simulink model "stackedRotor_dualEMRAX_dynInflow"  (R2022b)
settings: Solver=ode45  StartTime=0.0  StopTime=60  RelTol=1e-4  EnableMultiTasking=on
InitFcn:
  | %Hide scope plots
  | HidHandles = get(0,'ShowHiddenHandles');
  | set(0,'ShowHiddenHandles','On');
  | AllScopeHandles = findobj(0,'Type','Figure','Tag','SIMULINK_SIMSCOPE_FIGURE');
  | close(AllScopeHandles);
  | set(0,'ShowHiddenHandles',HidHandles);
  | 
  | %Load Cl and Cd from potential flow
  | load('C:\Users\msa2925\Box\Matt Lab Stuff\5th Year\Modeling\Look Up Tables\ClCd-1.mat');
  | 
  | %Load dynamic inflow properties (model and rotor_params)
  | load('C:\Users\msa2925\Box\Matt Lab Stuff\5th Year\Modeling\Look Up Tables\DynInflow-1.mat');
  | 
  | 
  | %Atmospheric Properties
  | rho_air    = 1.225;  % air density in kg/m^3
  | mu         = 1.803e-5; % dynamic viscosity [N-s/m^2]
  | 
  | %Emrax 208 Electrical Properties
  | R          = .0122;  %  resistance, ohms, line-line at room temp
  | L          = 125*10^-6;  %  inductance line-line at commutation frequency, henries
  | t_elec     = L/R;
  | Imotor     = 256/100^2;  %  kg*m^2 -- From Emrax data sheet
  | Kt_motor   = .80;  %  N*m/Arms
  | Ke_motor   = .0487*sqrt(2)*60/(2*pi);  %  Vpk/rad/sec
  | Ke         = .0487*sqrt(2)*60/(2*pi);   %radians/sec
  | POLES      = 20;
  | 
  | % no-load current fit (i0 = a1*omega^2 + a2) [Apk]
  | i_a1 = 8.98e-5;
  | i_a2 = 2.51;
  | 
  | %-----------Controller Properties------------------%
  | Vbus                 = 175;  % Actual bus voltage (volts) that will be applied
  | CurrentSenseMax      = 250;  %  Max current sense from controller code
  | BASE_CURRENT         = 125;   %  Max current in amps corresponding to normalized control loop current = 1
  | LOOP_FREQUENCY       = 35;     % orig: 35 in kHz
  | T_LOOP               = .001/LOOP_FREQUENCY;
  | pwm_loop_prescalar   = 1;  %Presacalar how many PWM cycles for one current loop execution
  | T_PWM                = T_LOOP/pwm_loop_prescalar;  %  Current loop prescaler on PWM is 1 for Uber
  | BASE_FREQ            = 1200; %POLES/2*1300/60;  %  1300 rpm
  | BaseSpeed            = BASE_FREQ*(60.0/(POLES/2.0));
  | omega                = 0;               % omega for de-coupling integrator
  | MsgFreq              = 1000; %Hz
  | 
  | %Current loop
  | alpha    = 250*2*pi;         % current loop bandwidth
  | I_Kp     = alpha*L*1;
  | I_Ki     = alpha*R/I_Kp*T_LOOP;
  | 
  | %Speed loop
  | SpeedLoopPrescale  = 5;
  | Tspeedloop         = T_LOOP*SpeedLoopPrescale;
  | PID_spd_Kp         = 4.75;   % From Uber code (ORIGINIAL: 3)
  | % PID_spd_Ki         = 2.1*Tspeedloop*1.5;   % From Uber code (ORIGINAL: 0.15*Tspeedloop*2)
  | PID_spd_Ki         = 1.75*Tspeedloop;
  | 
  | %Position loop
  | speedErrorPEngage    = .003; % Speed error max for position loop to enable
  | % Code has .001 for PEngage, trying something diff here
  | ... (+44 lines)
values from neighbouring files (symbols this model uses):
  AoA_sweep = [-2 -1 0 1 2 3 4 5 6 7 8 9 ... (13 elements, 1x13)]    [ClCd-1.mat]
  Cdl = [0.0123 0.0123 0.0123 0.0123 0.0123 0.0123 0.0123 0.0123 0.0123 0.0123 0.0123 0.0123 ... (6500 elements, 13x500)]    [ClCd-1.mat]
  Cdu = [0.0123 0.0123 0.0123 0.0123 0.0123 0.0123 0.0123 0.0123 0.0123 0.0123 0.0123 0.0123 ... (6500 elements, 13x500)]    [ClCd-1.mat]
  Cll = [-0.111113403346 0.00796289645531 0.127036770682 0.246071948277 0.365032169973 0.483881199334 0.602582833794 0.721100915686 0.839399343253 0.957442081649 1.07519317391 1.19261675192 ... (6500 elements, 13x500)]    [ClCd-1.mat]
  Clu = [-0.11705321178 0.00839337636768 0.133837407812 0.259240671085 0.384564967138 0.509772120977 0.634823993289 0.759682492064 0.884309584192 1.00866730705 1.13271778008 1.2564232163 ... (6500 elements, 13x500)]    [ClCd-1.mat]
  Cp = [0.000195201118563 0.000195344815163 0.000195970524669 0.000196911243155 0.000198292722473 0.000199793715635 0.000201836164013 0.000204359459521 0.00020706119236 0.00020992934584 0.000212955219574 0.000216131124695 ... (150 elements, 1x150)]    [BEMT-1.mat]    (also in BEMT-2.mat = [5.908e-05 5.908e-05 5.908e-05 5.908e-05 5.908e-05 5.908e-05; BEMT-3.mat = [6.167e-05 6.167e-05 6.167e-05 6.167e-05 6.167e-05 6.1671725; BEMT-PF-Isolated-1.mat = [6.88284627296e-05 6.76929537705e-05 6.92283244838e-05 7.518; BEMT-PF-Isolated-2.mat = [6.88286203447e-05 6.76929720507e-05 6.92293837373e-05 7.518)
  Cpl = [0.000333700998998 0.000390181039031 0.000394788670278 0.000400729506228 0.000408611755119 0.000419410254194 0.000434611180529 0.000454621522012 0.000471293145772 0.000468819202162 0.000461044856051 0.0004465872684 ... (37 elements, 1x37)]    [BEMT-PF-Stacked-1.mat]    (also in BEMT-PF-Stacked-3.mat = [0.00012095698162 0.000162284223538 0.000164817714818 0.0001; BEMT-PF-Stacked-4.mat = [0.000215313097577 0.00022323140747 0.000225181363314 0.0002; BEMT-PF-Stacked-5.mat = [0.000201399004141 0.000209364989981 0.000211223578331 0.000; CpData-Stacked-1.mat = [0.0004204989393 0.000429722690454 0.000432518606247 0.00043)
  Cpu = [0.000372640330495 0.000318761476241 0.00031503993434 0.000310316169544 0.000304143730405 0.000295773643033 0.00028387117424 0.000265492168428 0.000237641915024 0.000230728320611 0.000223594040333 0.000216887343718 ... (37 elements, 1x37)]    [BEMT-PF-Stacked-1.mat]    (also in BEMT-PF-Stacked-3.mat = [0.00014995136179 0.000108984048023 0.00010569458686 0.00010; BEMT-PF-Stacked-4.mat = [0.000200079302516 0.0001931098957 0.000191441123461 0.00018; BEMT-PF-Stacked-5.mat = [0.000223261524278 0.000214635121691 0.000212581398187 0.000; CpData-Stacked-1.mat = [0.000470292570894 0.000463315827435 0.000462372188797 0.000)
  Ct = [0 8.42066058624e-05 0.000168413211725 0.000252619817587 0.000348569118235 0.000435711397794 0.000522853677352 0.000609995956911 0.00069713823647 0.000784280516029 0.000871422795587 0.000958565075146 ... (150 elements, 1x150)]    [BEMT-1.mat]    (also in BEMT-2.mat = [-0.000241284312952 -0.00019885713846 -0.000156429963968 -0.; BEMT-3.mat = [-0.000252881464423 -0.00020500571035 -0.00015767832519 -0.0; BEMT-PF-Isolated-1.mat = [-0.000124730397385 6.78902114512e-07 0.000152796242494 0.00; BEMT-PF-Isolated-2.mat = [-0.000124743531158 6.68801957239e-07 0.000152879013625 0.00)
  Ctl = [0.00438668608339 0.0050628698524 0.00511522584539 0.00518172746808 0.00526807639226 0.00538256546486 0.00553531477508 0.00571551109899 0.00580582681419 0.00575766596858 0.00565748394784 0.00549586936617 ... (37 elements, 1x37)]    [BEMT-PF-Stacked-1.mat]    (also in BEMT-PF-Stacked-2.mat = [0.00446656952376 0.00504151525843 0.00508284852112 0.005134; BEMT-PF-Stacked-3.mat = [0.00184996435909 0.00209589101081 0.00210506301257 0.002127; BEMT-PF-Stacked-4.mat = [0.00305779502317 0.00317485141984 0.00320289061972 0.003237; BEMT-PF-Stacked-5.mat = [0.00284078729023 0.00295761000687 0.00298453442892 0.003017)
  Ctu = [0.00485875244254 0.00420098979139 0.00415434112966 0.00409491081367 0.00401692201007 0.00391066006909 0.00375881977479 0.00352379292731 0.0031675839941 0.00307949239151 0.00298865074931 0.00290335167779 ... (37 elements, 1x37)]    [BEMT-PF-Stacked-1.mat]    (also in BEMT-PF-Stacked-2.mat = [0.00487929290239 0.00430977798758 0.00426987840094 0.004219; BEMT-PF-Stacked-3.mat = [0.00202552929257 0.00178155832272 0.00175724958711 0.001735; BEMT-PF-Stacked-4.mat = [0.00282403441036 0.00271496837402 0.00268870985611 0.002655; BEMT-PF-Stacked-5.mat = [0.00315608603824 0.00303364263049 0.00300412792098 0.002966)
  index_sweep = [-90 -45 -40 -35 -30 -25 -20 -15 -10 -9 -8 -7 ... (37 elements, 1x37)]    [BEMT-PF-Stacked-1.mat]    (also in BEMT-PF-Stacked-2.mat; BEMT-PF-Stacked-3.mat = [-90 -45 -40 -35 -30 -25 -20 -15 -14 -13 -12 -11 ... (45 ele; BEMT-PF-Stacked-4.mat; BEMT-PF-Stacked-5.mat)
  index_sweep_Cp_table = [-90 -45.2679945682 -41.0748847617 -35.9788199136 -30.8261561384 -25.6873115637 -20.5477936424 -15.3629851439 -10.3005197032 -7.23856497031 -5.29357093665 -4.47027434572 ... (27 elements, 1x27)]    [CpData-Stacked-1.mat]
  model =     [DynInflow-1.mat]    (also in PP-1.mat; PP-2.mat; PP-3.mat)
  rotor_params =     [DynInflow-1.mat]    (also in PP-1.mat; PP-2.mat; PP-3.mat)
  theta = [-1.24244156171 -0.730247869575 -0.489791195362 -0.291308360013 -0.0904887039498 0.0775201787218 0.236938510902 0.389966557012 0.537998944025 0.680941129328 0.820002111662 0.955737387113 ... (150 elements, 1x150)]    [BEMT-1.mat]    (also in BEMT-2.mat = [-2.67472972391 -2.52181622329 -2.35655527709 -2.17339529035; BEMT-3.mat = [-2.61565298703 -2.45920727031 -2.29202818901 -2.11251263407; BEMT-PF-Isolated-1.mat = [-2 -1 0 1 2 3 4 5 6 7 8 9 ... (16 elements, 1x16)]; BEMT-PF-Isolated-2.mat = [-2 -1 0 1 2 3 4 5 6 7 8 9 ... (16 elements, 1x16)])
  x_sweep = [-1.74044233009 -1.73346660933 -1.72649088856 -1.7195151678 -1.71253944704 -1.70556372628 -1.69858800552 -1.69161228476 -1.68463656399 -1.67766084323 -1.67068512247 -1.66370940171 ... (500 elements, 1x500)]    [ClCd-1.mat]
undefined symbols (not defined in the file or in its folder): DiscIntNeverNeededParam
libraries: dspsrcs4 x2
(part 2 of 2)

== system stackedRotor_dualEMRAX_dynInflow/Follower/SVGEN-PWM ==
  note: Saturate to complex magnitude 1
  note: Output to PWM
      | after 11 us compute time
      | and wait for new PWM start
  note: Average V
      | across winding
      | takes 1 PWM
      | cycle to happen
  note: Compute
      | me
  DQ V : Inport
  Bus Voltage : Inport  Port=2
  Avg PWM voltage in DQ space : Product  RndMeth=Zero
  Complex to Magnitude-Angle : ComplexToMagnitudeAngle
  Complex to Real-Imag : ComplexToRealImag
  Conv to Cont time for Electical stuff : RateTransition
  Demux : Demux  Outputs=2
  Divide : Product  Inputs=/*
  Gain1 : Gain  Gain=1/sqrt(3)
  Into SVGEN : UnitDelay  InitialCondition=[ 0 ; omegamech*Ke/Vbus]  SampleTime=-1
  Magnitude-Angle to Complex : MagnitudeAngleToComplex
  Measure Bus V ADC : RateTransition  OutPortSampleTime=T_LOOP
  Mux : Mux  Inputs=2
  PWM emulation : RateTransition  OutPortSampleTime=T_PWM
  Real-Imag to Complex : RealImagToComplex
  Saturation : Saturate  UpperLimit=1  LowerLimit=-1
  Unit Delay : UnitDelay  InitialCondition=[ 0 ; omegamech*Ke/Vbus]  SampleTime=-1
  Unit Delay2 : UnitDelay  InitialCondition=[ 0 ; omegamech*Ke/Vbus]  SampleTime=-1
  DQ Volts : Outport
  wires:
  Into SVGEN/1 -> PWM emulation/1
  Unit Delay/1 -> Unit Delay2/1
  PWM emulation/1 -> Unit Delay/1
  Unit Delay2/1 -> Conv to Cont time for Electical stuff/1
  Bus Voltage/1 -> Gain1/1
  Measure Bus V ADC/1 -> Divide/1
  DQ V/1 -> Divide/2
  Conv to Cont time for Electical stuff/1 -> Avg PWM voltage in DQ space/2
  Avg PWM voltage in DQ space/1 -> DQ Volts/1
  Mux/1 -> Into SVGEN/1
  Divide/1 -> Demux/1
  Demux/1 -> Real-Imag to Complex/1
  Demux/2 -> Real-Imag to Complex/2
  Real-Imag to Complex/1 -> Complex to Magnitude-Angle/1
  Complex to Magnitude-Angle/1 -> Saturation/1
  Saturation/1 -> Magnitude-Angle to Complex/1
  Complex to Magnitude-Angle/2 -> Magnitude-Angle to Complex/2
  Magnitude-Angle to Complex/1 -> Complex to Real-Imag/1
  Complex to Real-Imag/1 -> Mux/1
  Complex to Real-Imag/2 -> Mux/2
  Gain1/1 -> Measure Bus V ADC/1, Avg PWM voltage in DQ space/1

== system stackedRotor_dualEMRAX_dynInflow/Follower/Speed Control? ==
  In1 : Inport
  Abs : Abs  SaturateOnIntegerOverflow=off
  Relay : Relay  OnSwitchValue=2*speedErrorPEngage  OffSwitchValue=speedErrorPEngage  OnOutputValue=0  OffOutputValue=1
  Out1 : Outport
  wires:
  Abs/1 -> Relay/1
  In1/1 -> Abs/1
  Relay/1 -> Out1/1

== system stackedRotor_dualEMRAX_dynInflow/Follower/Speed Controller ==
  In1 : Inport
  Initial Cond : Inport  Port=2
  Enable : EnablePort  ShowOutputPort=on
  1/integraltime to match code since Simulink integrator has Ts term : Gain  Gain=1/(T_LOOP*SpeedLoopPrescale)
  Add1 : Sum
  ControllerIN : Scope
  Discrete-Time Integrator : DiscreteIntegrator  InitialCondition=.03  SampleTime=-1  ICPrevOutput=DiscIntNeverNeededParam  ICPrevScaledInput=DiscIntNeverNeededParam
  Integrator term at the output : Gain  Gain=PID_spd_Kp
  Product : Product  RndMeth=Zero
  Product1 : Product  RndMeth=Zero
  Speed I gain : Constant  Value=PID_spd_Ki
  Speed P gain : Constant  Value=PID_spd_Kp
  Out1 : Outport
  State : Outport  Port=2
  wires:
  Product/1 -> 1/integraltime to match code since Simulink integrator has Ts term/1
  In1/1 -> Product/1, Add1/1
  1/integraltime to match code since Simulink integrator has Ts term/1 -> Discrete-Time Integrator/1
  Speed I gain/1 -> Product/2
  Speed P gain/1 -> Product1/1
  Discrete-Time Integrator/1 -> Integrator term at the output/1, ControllerIN/1, Add1/2
  Add1/1 -> Product1/2
  Product1/1 -> Out1/1
  Integrator term at the output/1 -> State/1

== system stackedRotor_dualEMRAX_dynInflow/Follower/Speed Estimator ==
  In1 : Inport
  Add1 : Sum  Inputs=+-
  DeltaAngle : Scope
  Sampling : UnitDelay  SampleTime=-1
  Speed Estimator : Subsystem
  Unit Delay1 : UnitDelay  SampleTime=-1
  Out1 : Outport
  wires:
  Sampling/1 -> Add1/1, Unit Delay1/1
  Unit Delay1/1 -> Add1/2
  Add1/1 -> Speed Estimator/1(delta angle), DeltaAngle/1
  In1/1 -> Sampling/1
  Speed Estimator/1(Est Speed [0,1]) -> Out1/1

== system stackedRotor_dualEMRAX_dynInflow/Follower/Wrap error2 ==
  In1 : Inport
  Add 2pi : Subsystem  TreatAsAtomicUnit=on
  If Action Subsystem : Subsystem  TreatAsAtomicUnit=on
  If1 : If  IfExpression=u1 > .5  ElseIfExpressions=u1<-.5
  Merge : Merge  Inputs=3
  Subtract 2pi1 : Subsystem  TreatAsAtomicUnit=on
  Out1 : Outport
  wires:
  In1/1 -> Add 2pi/1(In1), If Action Subsystem/1(In1), Subtract 2pi1/1(In1), If1/1
  Subtract 2pi1/1(Out1) -> Merge/1
  Merge/1 -> Out1/1
  If1/1 -> Subtract 2pi1/Action
  If1/3 -> If Action Subsystem/Action
  Add 2pi/1(Out1) -> Merge/2
  If Action Subsystem/1(Out1) -> Merge/3
  If1/2 -> Add 2pi/Action

== system stackedRotor_dualEMRAX_dynInflow/Servo/Angle Controller ==
  In1 : Inport
  Initial Cond : Inport  Port=2
  Enable1 : Inport  Port=3
  Angle Controller DT_PID saturate P : Subsystem
  Max error : Saturate  UpperLimit=PID_pos_error_sat  LowerLimit=-PID_pos_error_sat
  Out1 : Outport  InitialOutput=[0]
  State : Outport  Port=2  InitialOutput=[0]
  wires:
  Initial Cond/1 -> Angle Controller DT_PID saturate P/2(Iniitial Cond)
  Enable1/1 -> Angle Controller DT_PID saturate P/Enable
  Angle Controller DT_PID saturate P/1(Out1) -> Out1/1
  Angle Controller DT_PID saturate P/2(Integrator) -> State/1
  In1/1 -> Max error/1
  Max error/1 -> Angle Controller DT_PID saturate P/1(In1)

== system stackedRotor_dualEMRAX_dynInflow/Servo/Angle Error ==
  Revolution : Inport
  Commanded Rev : Inport  Port=2
  Add4 : Sum  Inputs=-+
  Angle Error Calc Deg : Scope
  Gain2 : Gain  Gain=360
  To Workspace3 : ToWorkspace  VariableName=Angle_err_servo  SaveFormat=Timeseries  SampleTime=-1
  Wrap error : Subsystem
  Revolution Error (norm) : Outport
  tag scope: angle_err_servo=global
  wires:
  Revolution/1 -> Add4/1
  Wrap error/1(Out1) -> [angle_err_servo], Revolution Error (norm)/1, Gain2/1
  Gain2/1 -> To Workspace3/1, Angle Error Calc Deg/1
  Add4/1 -> Wrap error/1(In1)
  Commanded Rev/1 -> Add4/2

== system stackedRotor_dualEMRAX_dynInflow/Servo/Current Controller ==
  note: D Current Reference
  note: D Current Feedback
  note: D Current Reference
  note: Q Current Reference
  note: Discrete
      | time control
      | law
  QI cmd : Inport
  DQ I feedback : Inport  Port=2
  Constant : Constant  Value=0
  Constant1 : Constant  Value=0
  D current PI controller : Subsystem
  Decoupling gain : Gain  Gain=alpha*omega*L
  Decoupling gain1 : Gain  Gain=alpha*omega*L
  Demux : Demux  Outputs=2
  Discrete-Time Integrator : DiscreteIntegrator  SampleTime=T_LOOP  ICPrevOutput=DiscIntNeverNeededParam  ICPrevScaledInput=DiscIntNeverNeededParam
  Discrete-Time Integrator1 : DiscreteIntegrator  SampleTime=T_LOOP  ICPrevOutput=DiscIntNeverNeededParam  ICPrevScaledInput=DiscIntNeverNeededParam
  Manual Switch : ManualSwitch
  Manual Switch1 : ManualSwitch  CurrentSetting=0
  Mux1 : Mux  Inputs=2
  Q current PI controller : Subsystem
  Sum2 : Sum  Inputs=|+-
  Sum3 : Sum  Inputs=|+-
  Sum5 : Sum  Inputs=|+-
  Sum6 : Sum  Inputs=++|
  DQ V cmd : Outport
  wires:
  Mux1/1 -> DQ V cmd/1
  Sum2/1 -> D current PI controller/1(In1), Manual Switch1/1
  Sum3/1 -> Q current PI controller/1(In1), Manual Switch/2
  Constant/1 -> Sum2/1
  D current PI controller/1(Out1) -> Sum5/1
  Q current PI controller/1(Out1) -> Sum6/2
  Discrete-Time Integrator/1 -> Sum6/1
  Discrete-Time Integrator1/1 -> Sum5/2
  QI cmd/1 -> Sum3/1
  Decoupling gain1/1 -> Discrete-Time Integrator1/1
  Decoupling gain/1 -> Discrete-Time Integrator/1
  Manual Switch/1 -> Decoupling gain1/1
  Manual Switch1/1 -> Decoupling gain/1
  Constant1/1 -> Manual Switch1/2, Manual Switch/1
  Sum5/1 -> Mux1/1
  Sum6/1 -> Mux1/2
  DQ I feedback/1 -> Demux/1
  Demux/1 -> Sum2/2
  Demux/2 -> Sum3/2

== system stackedRotor_dualEMRAX_dynInflow/Servo/Generate Angle vs time ==
  Speed : Inport
  Phase (norm) : Inport  Port=2
  Add5 : Sum
  Constant1 : Constant
  Constant3 : Constant
  Discrete-Time Integrator : DiscreteIntegrator  SampleTime=-1  ICPrevOutput=DiscIntNeverNeededParam  ICPrevScaledInput=DiscIntNeverNeededParam
  Normalized Mech Angle : Gain  Gain=BASE_FREQ/(POLES/2)
  Wrap command : Math  Operator=mod  SignedPower=on
  Wrap command1 : Math  Operator=mod  SignedPower=on
  Cmd Angle (norm) : Outport
  Reference Angle : Outport  Port=2
  wires:
  Constant1/1 -> Wrap command/2
  Discrete-Time Integrator/1 -> Normalized Mech Angle/1
  Add5/1 -> Wrap command/1
  Speed/1 -> Discrete-Time Integrator/1
  Phase (norm)/1 -> Add5/1
  Wrap command/1 -> Cmd Angle (norm)/1
  Constant3/1 -> Wrap command1/2
  Normalized Mech Angle/1 -> Wrap command1/1, Add5/2
  Wrap command1/1 -> Reference Angle/1

== system stackedRotor_dualEMRAX_dynInflow/Servo/Motor Efficiency ==
  note: Losses
  note: i0 fit
  I_eq : Inport
  omega_m : Inport  Port=2
  Constant1 : Constant  Value=i_a2
  Gain : Gain  Gain=i_a1
  IQ : Sum  Inputs=+-
  Kt : Gain  Gain=Kt_motor
  PL : Sum
  Pe : Sum
  Piron : Gain  Gain=Kt_motor
  Pm : Product
  Pres : Gain  Gain=3*R
  Product : Product
  Square : Math  Operator=square
  Square1 : Math  Operator=square
  eta_m : Product  Inputs=*/
  i0 : Sum
  Motor Efficiency : Outport
  Iq : Outport  Port=2
  wires:
  IQ/1 -> Iq/1, Kt/1
  Kt/1 -> Pm/1
  Pm/1 -> eta_m/1, Pe/1
  Pe/1 -> eta_m/2
  eta_m/1 -> Motor Efficiency/1
  Gain/1 -> i0/1
  Constant1/1 -> i0/2
  Square/1 -> Gain/1
  PL/1 -> Pe/2
  Pres/1 -> PL/1
  I_eq/1 -> Square1/1, IQ/1
  Square1/1 -> Pres/1
  omega_m/1 -> Product/1, Pm/2, Square/1
  Product/1 -> Piron/1
  Piron/1 -> PL/2
  i0/1 -> Product/2, IQ/2

== system stackedRotor_dualEMRAX_dynInflow/Servo/Motor Emag&winding ==
  note: Winding model
  DQ volts actual : Inport
  Motor Speed rad/sec : Inport  Port=2
  D Q currents : Scope
  Demux1 : Demux  Outputs=2
  Motor Back EMF : Gain  Gain=Ke_motor/sqrt(3)
  Mux2 : Mux  Inputs=2
  Subsystem : Subsystem
  Sum4 : Sum  Inputs=|+-
  DQ current : Outport
  wires:
  Motor Speed rad/sec/1 -> Motor Back EMF/1, Subsystem/2(Motor speed rad/sec)
  Mux2/1 -> Subsystem/1(DQ voltages)
  Demux1/1 -> Mux2/1
  Demux1/2 -> Sum4/1
  Sum4/1 -> Mux2/2
  Motor Back EMF/1 -> Sum4/2
  DQ volts actual/1 -> Demux1/1
  Subsystem/1(DQ currents) -> DQ current/1, D Q currents/1

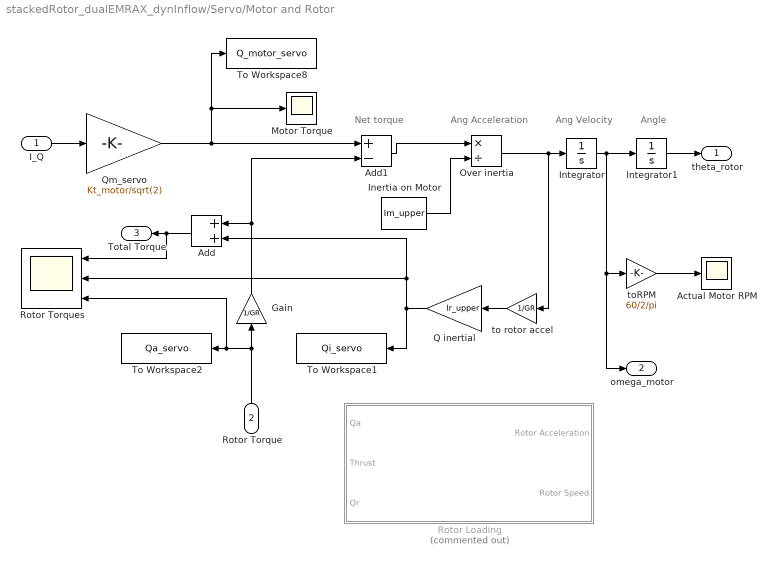
== system stackedRotor_dualEMRAX_dynInflow/Servo/Motor and Rotor ==
  note: Ang Acceleration
  note: Angle
  note: Ang Velocity
  note: Net torque
  I_Q : Inport
  Rotor Torque : Inport  Port=2
  Actual Motor RPM : Scope
  Add : Sum
  Add1 : Sum  Inputs=+-
  Gain : Gain  Gain=1/GR
  Inertia on Motor : Constant  Value=Im_upper
  Integrator : Integrator  InitialCondition=InitialRPM*2*pi/60
  Integrator1 : Integrator
  Motor Torque : Scope
  Over inertia : Product  Inputs=*/
  Q inertial : Gain  Gain=Ir_upper
  Qm_servo : Gain  Gain=Kt_motor/sqrt(2)
  Rotor Loading : Subsystem  Commented=on
  Rotor Torques : Scope  NumInputPorts=3
  To Workspace1 : ToWorkspace  VariableName=Qi_servo  SaveFormat=Timeseries  SampleTime=-1
  To Workspace2 : ToWorkspace  VariableName=Qa_servo  SaveFormat=Timeseries  SampleTime=-1
  To Workspace8 : ToWorkspace  VariableName=Q_motor_servo  SaveFormat=Timeseries  SampleTime=-1
  to rotor accel : Gain  Gain=1/GR
  toRPM : Gain  Gain=60/2/pi
  theta_rotor : Outport
  omega_motor : Outport  Port=2
  Total Torque : Outport  Port=3
  wires:
  Integrator/1 -> Integrator1/1, omega_motor/1, toRPM/1
  I_Q/1 -> Qm_servo/1
  Over inertia/1 -> to rotor accel/1, Integrator/1
  Integrator1/1 -> theta_rotor/1
  Add1/1 -> Over inertia/1
  toRPM/1 -> Actual Motor RPM/1
  to rotor accel/1 -> Q inertial/1
  Inertia on Motor/1 -> Over inertia/2
  Qm_servo/1 -> Motor Torque/1, To Workspace8/1, Add1/1
  Rotor Torque/1 -> Rotor Torques/3, To Workspace2/1, Gain/1
  Gain/1 -> Add/1, Add1/2
  Q inertial/1 -> Add/2, Rotor Torques/2, To Workspace1/1
  Add/1 -> Rotor Torques/1, Total Torque/1

== system stackedRotor_dualEMRAX_dynInflow/Servo/SVGEN-PWM ==
  note: Saturate to complex magnitude 1
  note: Output to PWM
      | after 11 us compute time
      | and wait for new PWM start
  note: Average V
      | across winding
      | takes 1 PWM
      | cycle to happen
  note: Compute
      | me
  DQ V : Inport
  Bus Voltage : Inport  Port=2
  Avg PWM voltage in DQ space : Product  RndMeth=Zero
  Complex to Magnitude-Angle : ComplexToMagnitudeAngle
  Complex to Real-Imag : ComplexToRealImag
  Conv to Cont time for Electical stuff : RateTransition
  Demux : Demux  Outputs=2
  Divide : Product  Inputs=/*
  Gain1 : Gain  Gain=1/sqrt(3)
  Into SVGEN : UnitDelay  InitialCondition=[ 0 ; omegamech*Ke/Vbus]  SampleTime=-1
  Magnitude-Angle to Complex : MagnitudeAngleToComplex
  Measure Bus V ADC : RateTransition  OutPortSampleTime=T_LOOP
  Mux : Mux  Inputs=2
  PWM emulation : RateTransition  OutPortSampleTime=T_PWM
  Real-Imag to Complex : RealImagToComplex
  Saturation : Saturate  UpperLimit=1  LowerLimit=-1
  Unit Delay : UnitDelay  InitialCondition=[ 0 ; omegamech*Ke/Vbus]  SampleTime=-1
  Unit Delay2 : UnitDelay  InitialCondition=[ 0 ; omegamech*Ke/Vbus]  SampleTime=-1
  DQ Volts : Outport
  wires:
  Into SVGEN/1 -> PWM emulation/1
  Unit Delay/1 -> Unit Delay2/1
  PWM emulation/1 -> Unit Delay/1
  Unit Delay2/1 -> Conv to Cont time for Electical stuff/1
  Bus Voltage/1 -> Gain1/1
  Measure Bus V ADC/1 -> Divide/1
  DQ V/1 -> Divide/2
  Conv to Cont time for Electical stuff/1 -> Avg PWM voltage in DQ space/2
  Avg PWM voltage in DQ space/1 -> DQ Volts/1
  Mux/1 -> Into SVGEN/1
  Divide/1 -> Demux/1
  Demux/1 -> Real-Imag to Complex/1
  Demux/2 -> Real-Imag to Complex/2
  Real-Imag to Complex/1 -> Complex to Magnitude-Angle/1
  Complex to Magnitude-Angle/1 -> Saturation/1
  Saturation/1 -> Magnitude-Angle to Complex/1
  Complex to Magnitude-Angle/2 -> Magnitude-Angle to Complex/2
  Magnitude-Angle to Complex/1 -> Complex to Real-Imag/1
  Complex to Real-Imag/1 -> Mux/1
  Complex to Real-Imag/2 -> Mux/2
  Gain1/1 -> Measure Bus V ADC/1, Avg PWM voltage in DQ space/1

== system stackedRotor_dualEMRAX_dynInflow/Servo/Speed Control? ==
  In1 : Inport
  Abs : Abs  SaturateOnIntegerOverflow=off
  Relay : Relay  OnSwitchValue=2*speedErrorPEngage  OffSwitchValue=speedErrorPEngage  OnOutputValue=0  OffOutputValue=1
  Out1 : Outport
  wires:
  Abs/1 -> Relay/1
  In1/1 -> Abs/1
  Relay/1 -> Out1/1

== system stackedRotor_dualEMRAX_dynInflow/Servo/Speed Controller ==
  In1 : Inport
  Initial Cond : Inport  Port=2
  Enable : EnablePort  ShowOutputPort=on
  1/integraltime to match code since Simulink integrator has Ts term : Gain  Gain=1/(T_LOOP*SpeedLoopPrescale)
  Add1 : Sum
  ControllerIN : Scope
  Discrete-Time Integrator : DiscreteIntegrator  InitialCondition=.03  SampleTime=-1  ICPrevOutput=DiscIntNeverNeededParam  ICPrevScaledInput=DiscIntNeverNeededParam
  Integrator term at the output : Gain  Gain=PID_spd_Kp
  Product : Product  RndMeth=Zero
  Product1 : Product  RndMeth=Zero
  Speed I gain : Constant  Value=PID_spd_Ki
  Speed P gain : Constant  Value=PID_spd_Kp
  Out1 : Outport
  State : Outport  Port=2
  wires:
  Product/1 -> 1/integraltime to match code since Simulink integrator has Ts term/1
  In1/1 -> Product/1, Add1/1
  1/integraltime to match code since Simulink integrator has Ts term/1 -> Discrete-Time Integrator/1
  Speed I gain/1 -> Product/2
  Speed P gain/1 -> Product1/1
  Discrete-Time Integrator/1 -> Integrator term at the output/1, ControllerIN/1, Add1/2
  Add1/1 -> Product1/2
  Product1/1 -> Out1/1
  Integrator term at the output/1 -> State/1

== system stackedRotor_dualEMRAX_dynInflow/Servo/Speed Estimator ==
  In1 : Inport
  Add1 : Sum  Inputs=+-
  DeltaAngle : Scope
  Sampling : UnitDelay  SampleTime=-1
  Speed Estimator : Subsystem
  Unit Delay1 : UnitDelay  SampleTime=-1
  Speed cmd : Outport
  wires:
  Sampling/1 -> Add1/1, Unit Delay1/1
  Unit Delay1/1 -> Add1/2
  Add1/1 -> Speed Estimator/1(delta angle), DeltaAngle/1
  In1/1 -> Sampling/1
  Speed Estimator/1(Est Speed [0,1]) -> Speed cmd/1

== system stackedRotor_dualEMRAX_dynInflow/Servo/Wrap error2 ==
  In1 : Inport
  Add 2pi : Subsystem  TreatAsAtomicUnit=on
  If Action Subsystem : Subsystem  TreatAsAtomicUnit=on
  If1 : If  IfExpression=u1 > .5  ElseIfExpressions=u1<-.5
  Merge : Merge  Inputs=3
  Subtract 2pi1 : Subsystem  TreatAsAtomicUnit=on
  Out1 : Outport
  wires:
  In1/1 -> Add 2pi/1(In1), If Action Subsystem/1(In1), Subtract 2pi1/1(In1), If1/1
  Subtract 2pi1/1(Out1) -> Merge/1
  Merge/1 -> Out1/1
  If1/1 -> Subtract 2pi1/Action
  If1/3 -> If Action Subsystem/Action
  Add 2pi/1(Out1) -> Merge/2
  If Action Subsystem/1(Out1) -> Merge/3
  If1/2 -> Add 2pi/Action

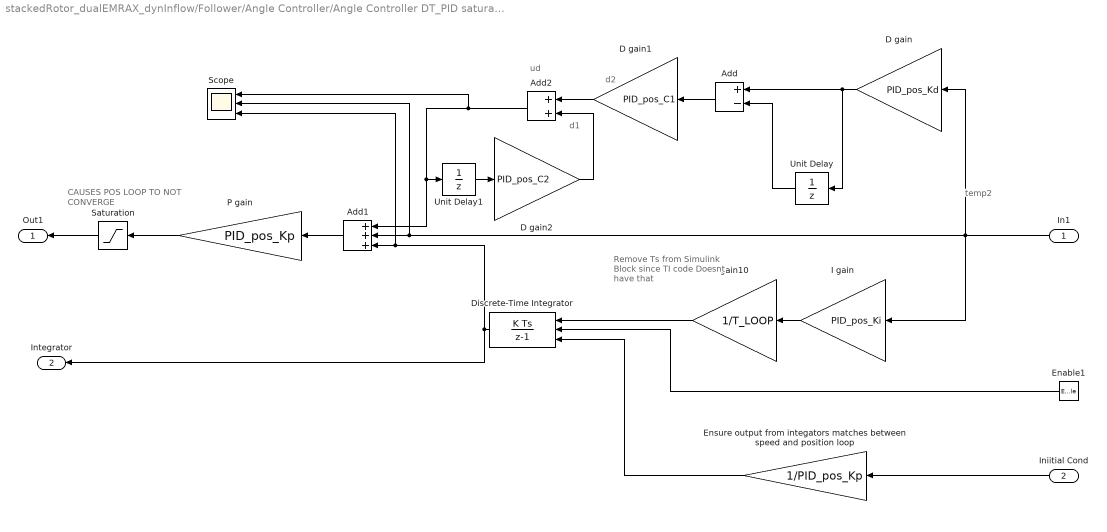
== system stackedRotor_dualEMRAX_dynInflow/Follower/Angle Controller/Angle Controller DT_PID saturate P ==
  note: CAUSES POS LOOP TO
      | NOT CONVERGE
  note: Remove Ts from Simulink
      | Block since TI code
      | Doesnt have that
  note: temp2
  note: d2
  note: ud
  note: d1
  In1 : Inport
  Iniitial Cond : Inport  Port=2
  Enable1 : EnablePort  ShowOutputPort=on
  Add : Sum  Inputs=+-
  Add1 : Sum  Inputs=+++
  Add2 : Sum
  D gain : Gain  Gain=PID_pos_Kd
  D gain1 : Gain  Gain=PID_pos_C1
  D gain2 : Gain  Gain=PID_pos_C2
  Discrete-Time Integrator : DiscreteIntegrator  ExternalReset=rising  InitialConditionSource=external  SampleTime=-1  UpperSaturationLimit=BASE_CURRENT  LowerSaturationLimit=-BASE_CURRENT  ICPrevOutput=DiscIntNeverNeededParam  ICPrevScaledInput=DiscIntNeverNeededParam
  Ensure output from integators matches between speed and position loop : Gain  Gain=1/PID_pos_Kp
  I gain : Gain  Gain=PID_pos_Ki
  P gain : Gain  Gain=PID_pos_Kp
  Saturation : Saturate  UpperLimit=PID_pos_sat  LowerLimit=-PID_pos_sat
  Scope : Scope  NumInputPorts=3
  Unit Delay : UnitDelay  SampleTime=-1
  Unit Delay1 : UnitDelay  SampleTime=-1
  gain10 : Gain  Gain=1/T_LOOP
  Out1 : Outport
  Integrator : Outport  Port=2
  wires:
  Discrete-Time Integrator/1 -> Scope/3, Add1/3, Integrator/1
  I gain/1 -> gain10/1
  In1/1 -> I gain/1, Scope/2, Add1/2, D gain/1
  Add1/1 -> P gain/1
  gain10/1 -> Discrete-Time Integrator/1
  Iniitial Cond/1 -> Ensure output from integators matches between speed and position loop/1
  Unit Delay/1 -> Add/2
  P gain/1 -> Saturation/1
  D gain/1 -> Add/1, Unit Delay/1
  Add/1 -> D gain1/1
  Unit Delay1/1 -> D gain2/1
  D gain2/1 -> Add2/2
  D gain1/1 -> Add2/1
  Ensure output from integators matches between speed and position loop/1 -> Discrete-Time Integrator/3
  Enable1/1 -> Discrete-Time Integrator/2
  Add2/1 -> Add1/1, Unit Delay1/1, Scope/1
  Saturation/1 -> Out1/1

== system stackedRotor_dualEMRAX_dynInflow/Follower/Angle Error/Wrap error ==
  In1 : Inport
  Add 2pi : Subsystem  TreatAsAtomicUnit=on
  If Action Subsystem : Subsystem  TreatAsAtomicUnit=on
  If1 : If  IfExpression=u1 > .5  ElseIfExpressions=u1<-.5
  Merge : Merge  Inputs=3
  Subtract 2pi1 : Subsystem  TreatAsAtomicUnit=on
  Out1 : Outport
  wires:
  In1/1 -> Add 2pi/1(In1), If Action Subsystem/1(In1), Subtract 2pi1/1(In1), If1/1
  Subtract 2pi1/1(Out1) -> Merge/1
  Merge/1 -> Out1/1
  If1/1 -> Subtract 2pi1/Action
  If1/3 -> If Action Subsystem/Action
  Add 2pi/1(Out1) -> Merge/2
  If Action Subsystem/1(Out1) -> Merge/3
  If1/2 -> Add 2pi/Action

== system stackedRotor_dualEMRAX_dynInflow/Follower/Current Controller/D current PI controller ==
  In1 : Inport
  Gain : Gain  Gain=I_Kp
  Gain1 : Gain  Gain=I_Ki
  K=1/Ts DT itegrator : DiscreteIntegrator  gainval=1/T_LOOP  InitialCondition=-2  SampleTime=-1  LimitOutput=on  UpperSaturationLimit=Vbus*sqrt(3)  LowerSaturationLimit=-Vbus*sqrt(3)  ICPrevOutput=DiscIntNeverNeededParam  ICPrevScaledInput=DiscIntNeverNeededParam
  Sum : Sum  Inputs=|++
  Out1 : Outport
  wires:
  In1/1 -> Gain/1
  Gain/1 -> Sum/1, Gain1/1
  Gain1/1 -> K=1/Ts DT itegrator/1
  K=1/Ts DT itegrator/1 -> Sum/2
  Sum/1 -> Out1/1

== system stackedRotor_dualEMRAX_dynInflow/Follower/Current Controller/Q current PI controller ==
  In1 : Inport
  1/Ts gain DT integrator : DiscreteIntegrator  gainval=1/T_LOOP  InitialCondition=80  SampleTime=-1  LimitOutput=on  UpperSaturationLimit=Vbus*sqrt(3)  LowerSaturationLimit=-Vbus*sqrt(3)  ICPrevOutput=DiscIntNeverNeededParam  ICPrevScaledInput=DiscIntNeverNeededParam
  Gain : Gain  Gain=I_Kp
  Gain1 : Gain  Gain=I_Ki
  Sum : Sum  Inputs=|++
  Out1 : Outport
  wires:
  Sum/1 -> Out1/1
  1/Ts gain DT integrator/1 -> Sum/2
  Gain1/1 -> 1/Ts gain DT integrator/1
  Gain/1 -> Sum/1, Gain1/1
  In1/1 -> Gain/1

== system stackedRotor_dualEMRAX_dynInflow/Follower/Motor Emag&winding/Subsystem ==
  DQ voltages : Inport
  Motor speed rad/sec : Inport  Port=2
  A : Concatenate  Mode=Multidimensional array
  Ax : Product  Multiplication=Matrix(*)  RndMeth=Zero
  Bu : Gain  Gain=2/L*[1 0 ; 0 1]  Multiplication=Matrix(K*u)
  Constant1 : Constant  Value=2/L*(-R/2)
  Constant2 : Constant  Value=2/L*(-R/2)
  Gain : Gain  Gain=-1
  Gain1 : Gain
  Integrator : Integrator  InitialCondition=[0 25]
  Matrix Concatenate : Concatenate  Mode=Multidimensional array  ConcatenateDimension=2
  Matrix Concatenate1 : Concatenate  Mode=Multidimensional array  ConcatenateDimension=2
  Sum : Sum
  To elec rad/sec : Gain  Gain=POLES/2
  DQ currents : Outport
  wires:
  DQ voltages/1 -> Bu/1
  Integrator/1 -> DQ currents/1, Ax/2
  Sum/1 -> Integrator/1
  Bu/1 -> Sum/1
  Motor speed rad/sec/1 -> To elec rad/sec/1
  Ax/1 -> Sum/2
  A/1 -> Ax/1
  Matrix Concatenate1/1 -> A/1
  Matrix Concatenate/1 -> A/2
  Constant1/1 -> Matrix Concatenate1/1
  Constant2/1 -> Matrix Concatenate/2
  Gain1/1 -> Matrix Concatenate1/2
  To elec rad/sec/1 -> Gain1/1, Gain/1
  Gain/1 -> Matrix Concatenate/1

== system stackedRotor_dualEMRAX_dynInflow/Follower/Motor and Rotor/Rotor Loading ==
  Rotor Acceleration : Inport
  Rotor Speed : Inport  Port=2
  1/GR : Gain  Gain=1/GR
  1/GR1 : Gain  Gain=1/GR
  Actual Prop RPM : Scope
  BEMT : Subsystem
  P inertial : Product  Inputs=**
  P total : Sum
  Q aero : Product  Inputs=*/
  Q inertial : Gain  Gain=Ir_lower
  Q total : Sum
  Rotor Powers : Scope  NumInputPorts=3
  Rotor Torques : Scope  NumInputPorts=3
  toRPM : Gain  Gain=60/2/pi
  Qa : Outport
  Thrust : Outport  Port=2
  Qr : Outport  Port=3
  wires:
  1/GR/1 -> Qa/1
  Q total/1 -> Rotor Torques/1, 1/GR1/1
  Q aero/1 -> 1/GR/1, Rotor Torques/3, Q total/2
  BEMT/1(P aero) -> Rotor Powers/3, P total/2, Q aero/1
  P total/1 -> Rotor Powers/1
  toRPM/1 -> Actual Prop RPM/1
  P inertial/1 -> P total/1, Rotor Powers/2
  Rotor Speed/1 -> BEMT/1(Rotor Speed), toRPM/1, Q aero/2, P inertial/2
  Q inertial/1 -> P inertial/1, Rotor Torques/2, Q total/1
  Rotor Acceleration/1 -> Q inertial/1
  BEMT/2(Thrust) -> Thrust/1
  1/GR1/1 -> Qr/1

== system stackedRotor_dualEMRAX_dynInflow/Follower/Speed Estimator/Speed Estimator ==
  delta angle : Inport
  Add1 : Sum  SampleTime=T_LOOP
  Filter gain for unity at 0 freq : Gain  Gain=K3
  Set filer pole : Gain  Gain=K2
  Unit Delay1 : UnitDelay  InitialCondition=.021  SampleTime=T_LOOP
  "[0,1] normalization unfiltered speed est from delta angle" : Gain  Gain=K1
  Est Speed [0,1] : Outport
  wires:
  delta angle/1 -> "[0,1] normalization unfiltered speed est from delta angle"/1
  Filter gain for unity at 0 freq/1 -> Add1/1
  Add1/1 -> Est Speed [0,1]/1, Unit Delay1/1
  Set filer pole/1 -> Add1/2
  Unit Delay1/1 -> Set filer pole/1
  "[0,1] normalization unfiltered speed est from delta angle"/1 -> Filter gain for unity at 0 freq/1

== system stackedRotor_dualEMRAX_dynInflow/Follower/Wrap error2/Add 2pi ==
  In1 : Inport
  Action Port : ActionPort  ActionPortLabel=elseif(u1<-.5)
  Add5 : Sum
  Constant2 : Constant
  Out1 : Outport
  wires:
  In1/1 -> Add5/1
  Add5/1 -> Out1/1
  Constant2/1 -> Add5/2

== system stackedRotor_dualEMRAX_dynInflow/Follower/Wrap error2/If Action Subsystem ==
  In1 : Inport
  Action Port : ActionPort  ActionPortLabel=else
  Out1 : Outport
  wires:
  In1/1 -> Out1/1

== system stackedRotor_dualEMRAX_dynInflow/Follower/Wrap error2/Subtract 2pi1 ==
  In1 : Inport
  Action Port : ActionPort  ActionPortLabel=if(u1 > .5)
  Add5 : Sum  Inputs=+-
  Constant2 : Constant
  Out1 : Outport
  wires:
  In1/1 -> Add5/1
  Add5/1 -> Out1/1
  Constant2/1 -> Add5/2

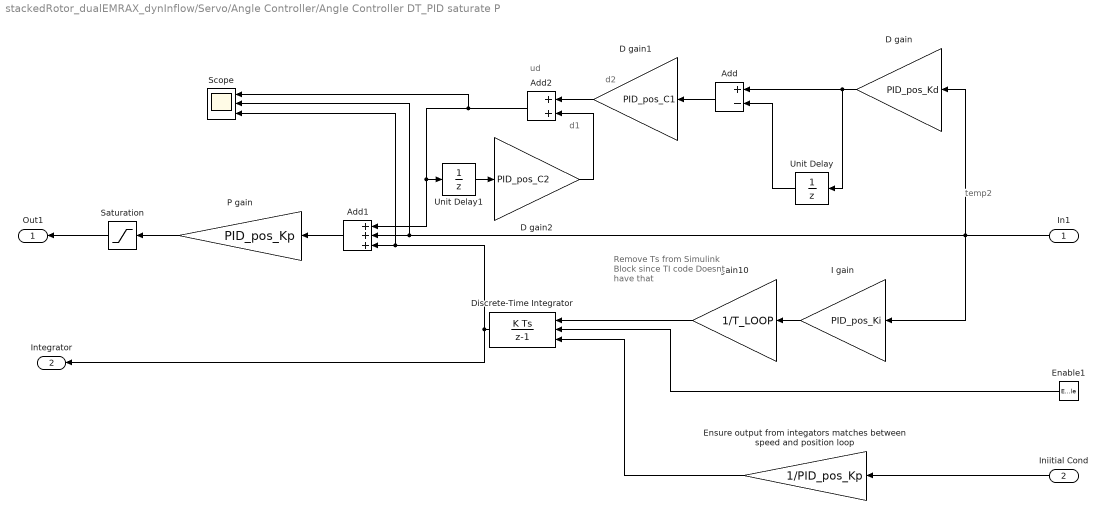
== system stackedRotor_dualEMRAX_dynInflow/Servo/Angle Controller/Angle Controller DT_PID saturate P ==
  note: Remove Ts from Simulink
      | Block since TI code
      | Doesnt have that
  note: temp2
  note: d2
  note: ud
  note: d1
  In1 : Inport
  Iniitial Cond : Inport  Port=2
  Enable1 : EnablePort  ShowOutputPort=on
  Add : Sum  Inputs=+-
  Add1 : Sum  Inputs=+++
  Add2 : Sum
  D gain : Gain  Gain=PID_pos_Kd
  D gain1 : Gain  Gain=PID_pos_C1
  D gain2 : Gain  Gain=PID_pos_C2
  Discrete-Time Integrator : DiscreteIntegrator  ExternalReset=rising  InitialConditionSource=external  SampleTime=-1  UpperSaturationLimit=BASE_CURRENT  LowerSaturationLimit=-BASE_CURRENT  ICPrevOutput=DiscIntNeverNeededParam  ICPrevScaledInput=DiscIntNeverNeededParam
  Ensure output from integators matches between speed and position loop : Gain  Gain=1/PID_pos_Kp
  I gain : Gain  Gain=PID_pos_Ki
  P gain : Gain  Gain=PID_pos_Kp
  Saturation : Saturate  UpperLimit=PID_pos_sat  LowerLimit=-PID_pos_sat
  Scope : Scope  NumInputPorts=3
  Unit Delay : UnitDelay  SampleTime=-1
  Unit Delay1 : UnitDelay  SampleTime=-1
  gain10 : Gain  Gain=1/T_LOOP
  Out1 : Outport
  Integrator : Outport  Port=2
  wires:
  Discrete-Time Integrator/1 -> Scope/3, Add1/3, Integrator/1
  I gain/1 -> gain10/1
  In1/1 -> I gain/1, Scope/2, Add1/2, D gain/1
  Add1/1 -> P gain/1
  gain10/1 -> Discrete-Time Integrator/1
  Iniitial Cond/1 -> Ensure output from integators matches between speed and position loop/1
  Unit Delay/1 -> Add/2
  P gain/1 -> Saturation/1
  D gain/1 -> Add/1, Unit Delay/1
  Add/1 -> D gain1/1
  Unit Delay1/1 -> D gain2/1
  D gain2/1 -> Add2/2
  D gain1/1 -> Add2/1
  Ensure output from integators matches between speed and position loop/1 -> Discrete-Time Integrator/3
  Enable1/1 -> Discrete-Time Integrator/2
  Add2/1 -> Add1/1, Unit Delay1/1, Scope/1
  Saturation/1 -> Out1/1

== system stackedRotor_dualEMRAX_dynInflow/Servo/Angle Error/Wrap error ==
  In1 : Inport
  Add 2pi : Subsystem  TreatAsAtomicUnit=on
  If Action Subsystem : Subsystem  TreatAsAtomicUnit=on
  If1 : If  IfExpression=u1 > .5  ElseIfExpressions=u1<-.5
  Merge : Merge  Inputs=3
  Subtract 2pi1 : Subsystem  TreatAsAtomicUnit=on
  Out1 : Outport
  wires:
  In1/1 -> Add 2pi/1(In1), If Action Subsystem/1(In1), Subtract 2pi1/1(In1), If1/1
  Subtract 2pi1/1(Out1) -> Merge/1
  Merge/1 -> Out1/1
  If1/1 -> Subtract 2pi1/Action
  If1/3 -> If Action Subsystem/Action
  Add 2pi/1(Out1) -> Merge/2
  If Action Subsystem/1(Out1) -> Merge/3
  If1/2 -> Add 2pi/Action

== system stackedRotor_dualEMRAX_dynInflow/Servo/Current Controller/D current PI controller ==
  In1 : Inport
  Gain : Gain  Gain=I_Kp
  Gain1 : Gain  Gain=I_Ki
  K=1/Ts DT itegrator : DiscreteIntegrator  gainval=1/T_LOOP  InitialCondition=-2  SampleTime=-1  LimitOutput=on  UpperSaturationLimit=Vbus*sqrt(3)  LowerSaturationLimit=-Vbus*sqrt(3)  ICPrevOutput=DiscIntNeverNeededParam  ICPrevScaledInput=DiscIntNeverNeededParam
  Sum : Sum  Inputs=|++
  Out1 : Outport
  wires:
  In1/1 -> Gain/1
  Gain/1 -> Sum/1, Gain1/1
  Gain1/1 -> K=1/Ts DT itegrator/1
  K=1/Ts DT itegrator/1 -> Sum/2
  Sum/1 -> Out1/1

== system stackedRotor_dualEMRAX_dynInflow/Servo/Current Controller/Q current PI controller ==
  In1 : Inport
  1/Ts gain DT integrator : DiscreteIntegrator  gainval=1/T_LOOP  InitialCondition=80  SampleTime=-1  LimitOutput=on  UpperSaturationLimit=Vbus*sqrt(3)  LowerSaturationLimit=-Vbus*sqrt(3)  ICPrevOutput=DiscIntNeverNeededParam  ICPrevScaledInput=DiscIntNeverNeededParam
  Gain : Gain  Gain=I_Kp
  Gain1 : Gain  Gain=I_Ki
  Sum : Sum  Inputs=|++
  Out1 : Outport
  wires:
  Sum/1 -> Out1/1
  1/Ts gain DT integrator/1 -> Sum/2
  Gain1/1 -> 1/Ts gain DT integrator/1
  Gain/1 -> Sum/1, Gain1/1
  In1/1 -> Gain/1

== system stackedRotor_dualEMRAX_dynInflow/Servo/Motor Emag&winding/Subsystem ==
  DQ voltages : Inport
  Motor speed rad/sec : Inport  Port=2
  A : Concatenate  Mode=Multidimensional array
  Ax : Product  Multiplication=Matrix(*)  RndMeth=Zero
  Bu : Gain  Gain=2/L*[1 0 ; 0 1]  Multiplication=Matrix(K*u)
  Constant1 : Constant  Value=2/L*(-R/2)
  Constant2 : Constant  Value=2/L*(-R/2)
  Gain : Gain  Gain=-1
  Gain1 : Gain
  Integrator : Integrator  InitialCondition=[0 25]
  Matrix Concatenate : Concatenate  Mode=Multidimensional array  ConcatenateDimension=2
  Matrix Concatenate1 : Concatenate  Mode=Multidimensional array  ConcatenateDimension=2
  Sum : Sum
  To elec rad/sec : Gain  Gain=POLES/2
  DQ currents : Outport
  wires:
  DQ voltages/1 -> Bu/1
  Integrator/1 -> DQ currents/1, Ax/2
  Sum/1 -> Integrator/1
  Bu/1 -> Sum/1
  Motor speed rad/sec/1 -> To elec rad/sec/1
  Ax/1 -> Sum/2
  A/1 -> Ax/1
  Matrix Concatenate1/1 -> A/1
  Matrix Concatenate/1 -> A/2
  Constant1/1 -> Matrix Concatenate1/1
  Constant2/1 -> Matrix Concatenate/2
  Gain1/1 -> Matrix Concatenate1/2
  To elec rad/sec/1 -> Gain1/1, Gain/1
  Gain/1 -> Matrix Concatenate/1

== system stackedRotor_dualEMRAX_dynInflow/Servo/Motor and Rotor/Rotor Loading ==
  Rotor Acceleration : Inport
  Rotor Speed : Inport  Port=2
  1/GR : Gain  Gain=1/GR
  1/GR1 : Gain  Gain=1/GR
  Actual Prop RPM : Scope
  BEMT : Subsystem
  P inertial : Product  Inputs=**
  P total : Sum
  Q aero : Product  Inputs=*/
  Q inertial : Gain  Gain=Ir_upper
  Q total : Sum
  Rotor Powers : Scope  NumInputPorts=3
  Rotor Torques : Scope  NumInputPorts=3
  toRPM : Gain  Gain=60/2/pi
  Qa : Outport
  Thrust : Outport  Port=2
  Qr : Outport  Port=3
  wires:
  1/GR/1 -> Qa/1
  Q total/1 -> Rotor Torques/1, 1/GR1/1
  Q aero/1 -> 1/GR/1, Rotor Torques/3, Q total/2
  BEMT/1(P aero) -> Rotor Powers/3, P total/2, Q aero/1
  P total/1 -> Rotor Powers/1
  toRPM/1 -> Actual Prop RPM/1
  P inertial/1 -> P total/1, Rotor Powers/2
  Rotor Speed/1 -> Q aero/2, P inertial/2, BEMT/1(Rotor Speed), toRPM/1
  Q inertial/1 -> Rotor Torques/2, Q total/1, P inertial/1
  Rotor Acceleration/1 -> Q inertial/1
  BEMT/2(Thrust) -> Thrust/1
  1/GR1/1 -> Qr/1

== system stackedRotor_dualEMRAX_dynInflow/Servo/Speed Estimator/Speed Estimator ==
  delta angle : Inport
  Add1 : Sum  SampleTime=T_LOOP
  Filter gain for unity at 0 freq : Gain  Gain=K3
  Set filer pole : Gain  Gain=K2
  Unit Delay1 : UnitDelay  InitialCondition=.021  SampleTime=T_LOOP
  "[0,1] normalization unfiltered speed est from delta angle" : Gain  Gain=K1
  Est Speed [0,1] : Outport
  wires:
  delta angle/1 -> "[0,1] normalization unfiltered speed est from delta angle"/1
  Filter gain for unity at 0 freq/1 -> Add1/1
  Add1/1 -> Est Speed [0,1]/1, Unit Delay1/1
  Set filer pole/1 -> Add1/2
  Unit Delay1/1 -> Set filer pole/1
  "[0,1] normalization unfiltered speed est from delta angle"/1 -> Filter gain for unity at 0 freq/1

== system stackedRotor_dualEMRAX_dynInflow/Servo/Wrap error2/Add 2pi ==
  In1 : Inport
  Action Port : ActionPort  ActionPortLabel=elseif(u1<-.5)
  Add5 : Sum
  Constant2 : Constant
  Out1 : Outport
  wires:
  In1/1 -> Add5/1
  Add5/1 -> Out1/1
  Constant2/1 -> Add5/2

== system stackedRotor_dualEMRAX_dynInflow/Servo/Wrap error2/If Action Subsystem ==
  In1 : Inport
  Action Port : ActionPort  ActionPortLabel=else
  Out1 : Outport
  wires:
  In1/1 -> Out1/1

== system stackedRotor_dualEMRAX_dynInflow/Servo/Wrap error2/Subtract 2pi1 ==
  In1 : Inport
  Action Port : ActionPort  ActionPortLabel=if(u1 > .5)
  Add5 : Sum  Inputs=+-
  Constant2 : Constant
  Out1 : Outport
  wires:
  In1/1 -> Add5/1
  Add5/1 -> Out1/1
  Constant2/1 -> Add5/2

== system stackedRotor_dualEMRAX_dynInflow/Follower/Angle Error/Wrap error/Add 2pi ==
  In1 : Inport
  Action Port : ActionPort  ActionPortLabel=elseif(u1<-.5)
  Add5 : Sum
  Constant2 : Constant
  Out1 : Outport
  wires:
  In1/1 -> Add5/1
  Add5/1 -> Out1/1
  Constant2/1 -> Add5/2

== system stackedRotor_dualEMRAX_dynInflow/Follower/Angle Error/Wrap error/If Action Subsystem ==
  In1 : Inport
  Action Port : ActionPort  ActionPortLabel=else
  Out1 : Outport
  wires:
  In1/1 -> Out1/1

== system stackedRotor_dualEMRAX_dynInflow/Follower/Angle Error/Wrap error/Subtract 2pi1 ==
  In1 : Inport
  Action Port : ActionPort  ActionPortLabel=if(u1 > .5)
  Add5 : Sum  Inputs=+-
  Constant2 : Constant
  Out1 : Outport
  wires:
  In1/1 -> Add5/1
  Add5/1 -> Out1/1
  Constant2/1 -> Add5/2

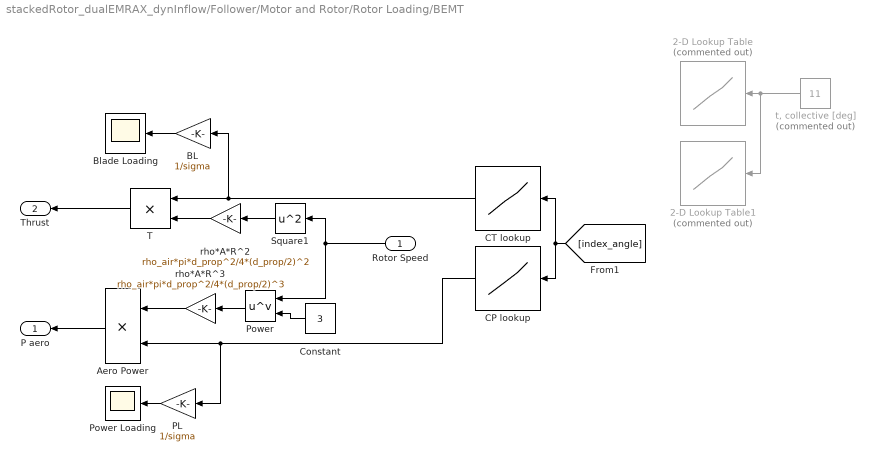
== system stackedRotor_dualEMRAX_dynInflow/Follower/Motor and Rotor/Rotor Loading/BEMT ==
  Rotor Speed : Inport
  2-D Lookup Table : Lookup_n-D  Commented=on  NumberOfTableDimensions=1  BreakpointsForDimension1=theta  BreakpointsForDimension2=[1:3]  Table=Ct  InternalRulePriority=Speed  RndMeth=Simplest
  2-D Lookup Table1 : Lookup_n-D  Commented=on  NumberOfTableDimensions=1  BreakpointsForDimension1=theta  BreakpointsForDimension2=[1:3]  Table=Cp  InternalRulePriority=Speed  RndMeth=Simplest
  Aero Power : Product  Inputs=**
  BL : Gain  Gain=1/sigma
  Blade Loading : Scope
  CP lookup : Lookup_n-D  NumberOfTableDimensions=1  BreakpointsForDimension1=index_sweep_Cp_table  BreakpointsForDimension2=[1:3]  Table=Cpl  InternalRulePriority=Speed  RndMeth=Simplest
  CT lookup : Lookup_n-D  NumberOfTableDimensions=1  BreakpointsForDimension1=index_sweep  BreakpointsForDimension2=[1:3]  Table=Ctl  InternalRulePriority=Speed  RndMeth=Simplest
  Constant : Constant  Value=3
  PL : Gain  Gain=1/sigma
  Power : Math  Operator=pow
  Power Loading : Scope
  Square1 : Math  Operator=square
  T : Product  Inputs=**
  rho*A*R^2 : Gain  Gain=rho_air*pi*d_prop^2/4*(d_prop/2)^2
  rho*A*R^3 : Gain  Gain=rho_air*pi*d_prop^2/4*(d_prop/2)^3
  "t, collective [deg]" : Constant  Commented=on  Value=11
  P aero : Outport
  Thrust : Outport  Port=2
  wires:
  rho*A*R^3/1 -> Aero Power/1
  Rotor Speed/1 -> Power/1, Square1/1
  Power/1 -> rho*A*R^3/1
  Square1/1 -> rho*A*R^2/1
  Aero Power/1 -> P aero/1
  BL/1 -> Blade Loading/1
  T/1 -> Thrust/1
  Constant/1 -> Power/2
  "t, collective [deg]"/1 -> 2-D Lookup Table1/1, 2-D Lookup Table/1
  CP lookup/1 -> PL/1, Aero Power/2
  CT lookup/1 -> T/1, BL/1
  rho*A*R^2/1 -> T/2
  PL/1 -> Power Loading/1
  [index_angle] -> CP lookup/1, CT lookup/1

== system stackedRotor_dualEMRAX_dynInflow/Servo/Angle Error/Wrap error/Add 2pi ==
  In1 : Inport
  Action Port : ActionPort  ActionPortLabel=elseif(u1<-.5)
  Add5 : Sum
  Constant2 : Constant
  Out1 : Outport
  wires:
  In1/1 -> Add5/1
  Add5/1 -> Out1/1
  Constant2/1 -> Add5/2

== system stackedRotor_dualEMRAX_dynInflow/Servo/Angle Error/Wrap error/If Action Subsystem ==
  In1 : Inport
  Action Port : ActionPort  ActionPortLabel=else
  Out1 : Outport
  wires:
  In1/1 -> Out1/1

== system stackedRotor_dualEMRAX_dynInflow/Servo/Angle Error/Wrap error/Subtract 2pi1 ==
  In1 : Inport
  Action Port : ActionPort  ActionPortLabel=if(u1 > .5)
  Add5 : Sum  Inputs=+-
  Constant2 : Constant
  Out1 : Outport
  wires:
  In1/1 -> Add5/1
  Add5/1 -> Out1/1
  Constant2/1 -> Add5/2

== system stackedRotor_dualEMRAX_dynInflow/Servo/Motor and Rotor/Rotor Loading/BEMT ==
  Rotor Speed : Inport
  2-D Lookup Table : Lookup_n-D  Commented=on  NumberOfTableDimensions=1  BreakpointsForDimension1=theta  BreakpointsForDimension2=[1:3]  Table=Ct  InternalRulePriority=Speed  RndMeth=Simplest
  2-D Lookup Table1 : Lookup_n-D  Commented=on  NumberOfTableDimensions=1  BreakpointsForDimension1=theta  BreakpointsForDimension2=[1:3]  Table=Cp  InternalRulePriority=Speed  RndMeth=Simplest
  Aero Power : Product  Inputs=**
  BL : Gain  Gain=1/sigma
  Blade Loading : Scope
  CP lookup : Lookup_n-D  NumberOfTableDimensions=1  BreakpointsForDimension1=index_sweep_Cp_table  BreakpointsForDimension2=[1:3]  Table=Cpu  InternalRulePriority=Speed  RndMeth=Simplest
  CT lookup : Lookup_n-D  NumberOfTableDimensions=1  BreakpointsForDimension1=index_sweep  BreakpointsForDimension2=[1:3]  Table=Ctu  InternalRulePriority=Speed  RndMeth=Simplest
  Constant : Constant  Value=3
  PL : Gain  Gain=1/sigma
  Power : Math  Operator=pow
  Power Loading : Scope
  Square1 : Math  Operator=square
  T : Product  Inputs=**
  rho*A*R^2 : Gain  Gain=rho_air*pi*d_prop^2/4*(d_prop/2)^2
  rho*A*R^3 : Gain  Gain=rho_air*pi*d_prop^2/4*(d_prop/2)^3
  "t, collective [deg]" : Constant  Commented=on  Value=11
  P aero : Outport
  Thrust : Outport  Port=2
  wires:
  rho*A*R^3/1 -> Aero Power/1
  Rotor Speed/1 -> Power/1, Square1/1
  Power/1 -> rho*A*R^3/1
  Square1/1 -> rho*A*R^2/1
  Aero Power/1 -> P aero/1
  BL/1 -> Blade Loading/1
  T/1 -> Thrust/1
  Constant/1 -> Power/2
  "t, collective [deg]"/1 -> 2-D Lookup Table1/1, 2-D Lookup Table/1
  CP lookup/1 -> PL/1, Aero Power/2
  CT lookup/1 -> T/1, BL/1
  rho*A*R^2/1 -> T/2
  PL/1 -> Power Loading/1
  ? -> CT lookup/1, CP lookup/1
